simulink model "Six_DOF"  (R2017a)
settings: Solver=ode45  StartTime=0.0  StopTime=10  MaxStep=2.0  RelTol=1e-3
InitFcn:
  | initializeVariables
StopFcn:
  | postProcessResults
undefined symbols (not defined in the file): airplane, cl_fit, cm_fit, cx_fit, m
libraries: simulink_extras x5, aerolibasang x3, shared6dof x1
settings Model: Creator=Devansh  LastModifiedBy=Devansh
settings HardwareCC: ProdBitPerLong=64  ProdHWDeviceType=Intel->x86-64 (Mac OS X)

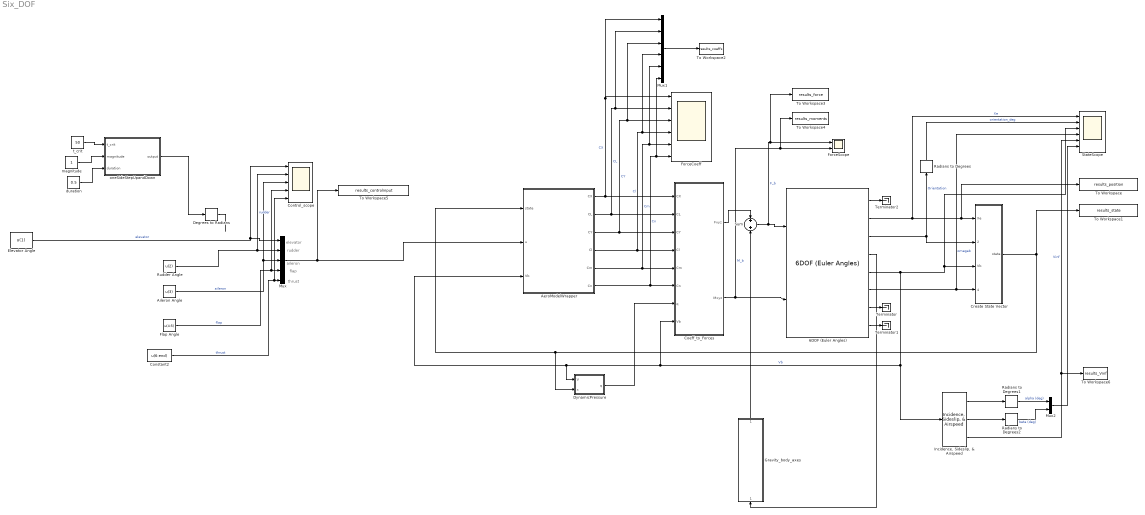
== system Six_DOF ==
  note: thrust
  note: flap
  note: aileron
  note: rudder
  note: elevator
  6DOF (Euler Angles) : shared6dof/6DOF (Euler Angles)  units=Metric (MKS)  mtype=Fixed  rep=Euler Angles  xme_0=initial_position  Vm_0=initial_velocity  eul_0=initial_orientation  pm_0=initial_rotation_rate  mass_0=m  mass_e=0.5  mass_f=2.0  inertia=inertia_matrix  inertia_e=eye(3)  inertia_f=2*eye(3)  k_quat=1.0  vre_flag=on  abi_flag=off
  AeroModelWrapper : Subsystem
  Aileron Angle : Constant  Value=u(3)
  Coeff_to_Forces : Subsystem  TreatAsAtomicUnit=on
  Constant2 : Constant  Value=u(6:end)
  Control_scope : Scope  NumInputPorts=5
  Create State Vector : Subsystem
  Degrees to Radians : simulink_extras/Transformations/Degrees to Radians
  DynamicPressure : MATLAB Function  TreatAsAtomicUnit=on
  Elevator Angle : Constant  Value=u(1)
  Flap Angle : Constant  Value=u(4:5)
  ForceCoeff : Scope  NumInputPorts=6
  ForceScope : Scope  NumInputPorts=2
  Gravity_body_axes : Subsystem
  "Incidence, Sideslip, & Airspeed" : aerolibasang/Incidence, Sideslip, & Airspeed
      settings: SourceProductName=Aerospace Blockset
  Mux : Mux  Inputs=5
  Mux1 : Mux  Inputs=6
  Mux2 : Mux  Inputs=2
  Radians to Degrees : simulink_extras/Transformations/Radians to Degrees
  Radians to Degrees1 : simulink_extras/Transformations/Radians to Degrees
  Radians to Degrees2 : simulink_extras/Transformations/Radians to Degrees
  Rudder Angle : Constant  Value=u(2)
  "StateScope " : Scope  NumInputPorts=6
  Sum : Sum  Inputs=+|+
  Terminator : Terminator
  Terminator1 : Terminator
  Terminator2 : Terminator
  To Workspace : ToWorkspace  VariableName=results_position  SaveFormat=Timeseries  SampleTime=-1
  To Workspace1 : ToWorkspace  VariableName=results_state  SaveFormat=Timeseries  SampleTime=-1
  To Workspace2 : ToWorkspace  VariableName=results_coeffs  SaveFormat=Timeseries  SampleTime=-1
  To Workspace3 : ToWorkspace  VariableName=results_force  SaveFormat=Timeseries  SampleTime=-1
  To Workspace4 : ToWorkspace  VariableName=results_moments  SaveFormat=Timeseries  SampleTime=-1
  To Workspace5 : ToWorkspace  VariableName=results_controlinput  SaveFormat=Timeseries  SampleTime=-1
  To Workspace6 : ToWorkspace  VariableName=results_Vinf  SaveFormat=Timeseries  SampleTime=-1
  duration : Constant  Value=0.5
  magnitude : Constant
  oneSideStepUpandDown : Subsystem
  t_crit : Constant  Value=50
  wires:
  AeroModelWrapper/1(CX) -> Coeff_to_Forces/1(CX), Mux1/1, ForceCoeff/1  "CX"
  AeroModelWrapper/3(CY) -> Coeff_to_Forces/3(CY), Mux1/3, ForceCoeff/3  "CY"
  AeroModelWrapper/2(CL) -> Coeff_to_Forces/2(CL), Mux1/2, ForceCoeff/2  "CL"
  AeroModelWrapper/4(Cl) -> Mux1/4, ForceCoeff/4, Coeff_to_Forces/4(Cl)  "Cl"
  AeroModelWrapper/5(Cm) -> Mux1/5, ForceCoeff/5, Coeff_to_Forces/5(Cm)  "Cm"
  AeroModelWrapper/6(Cn) -> Mux1/6, ForceCoeff/6, Coeff_to_Forces/6(Cn)  "Cn"
  Coeff_to_Forces/2(Mxyz) -> To Workspace4/1, ForceScope/2, 6DOF (Euler Angles)/2  "M_b"
  DynamicPressure/1(q) -> Coeff_to_Forces/7(q)
  6DOF (Euler Angles)/2 -> "StateScope "/1, To Workspace/1, Create State Vector/1(Xe)  "Xe"
  6DOF (Euler Angles)/3 -> Create State Vector/2(orientation), Radians to Degrees/1  "Orientation"
  6DOF (Euler Angles)/5 -> "StateScope "/3, Create State Vector/3(Vb), "Incidence, Sideslip, & Airspeed"/1, Coeff_to_Forces/8(Vb), AeroModelWrapper/3(Vb), DynamicPressure/1(V)  "Vb"
  6DOF (Euler Angles)/6 -> "StateScope "/4, Create State Vector/4(omega b)  "omegab"
  Flap Angle/1 -> Control_scope/4, Mux/4  "flap"
  Constant2/1 -> Control_scope/5, Mux/5  "thrust"
  "Incidence, Sideslip, & Airspeed"/3 -> "StateScope "/5, To Workspace6/1  "Vinf"
  "Incidence, Sideslip, & Airspeed"/1 -> Radians to Degrees1/1
  "Incidence, Sideslip, & Airspeed"/2 -> Radians to Degrees2/1
  Radians to Degrees/1 -> "StateScope "/2  "orientation_deg"
  Radians to Degrees1/1 -> Mux2/1  "alpha (deg)"
  Radians to Degrees2/1 -> Mux2/2  "beta (deg)"
  Coeff_to_Forces/1(Fxyz) -> Sum/1
  Sum/1 -> 6DOF (Euler Angles)/1, To Workspace3/1, ForceScope/1  "F_b"
  6DOF (Euler Angles)/4 -> Gravity_body_axes/1(Earth_to_body_rotation)
  Gravity_body_axes/1(Gravity_Body_coords) -> Sum/2
  Mux/1 -> To Workspace5/1, AeroModelWrapper/2(u)
  6DOF (Euler Angles)/7 -> Terminator/1
  6DOF (Euler Angles)/8 -> Terminator1/1
  6DOF (Euler Angles)/1 -> Terminator2/1
  Degrees to Radians/1 -> ?
  t_crit/1 -> oneSideStepUpandDown/1(t_crit)
  magnitude/1 -> oneSideStepUpandDown/2(magnitude)
  duration/1 -> oneSideStepUpandDown/3(duration)
  oneSideStepUpandDown/1(output) -> Degrees to Radians/1
  Elevator Angle/1 -> Control_scope/1, Mux/1  "elevator"
  Rudder Angle/1 -> Control_scope/2, Mux/2  "rudder"
  Aileron Angle/1 -> Control_scope/3, Mux/3  "aileron"
  Mux1/1 -> To Workspace2/1
  Create State Vector/1(state) -> To Workspace1/1, DynamicPressure/2(x), AeroModelWrapper/1(state)
  Mux2/1 -> "StateScope "/6

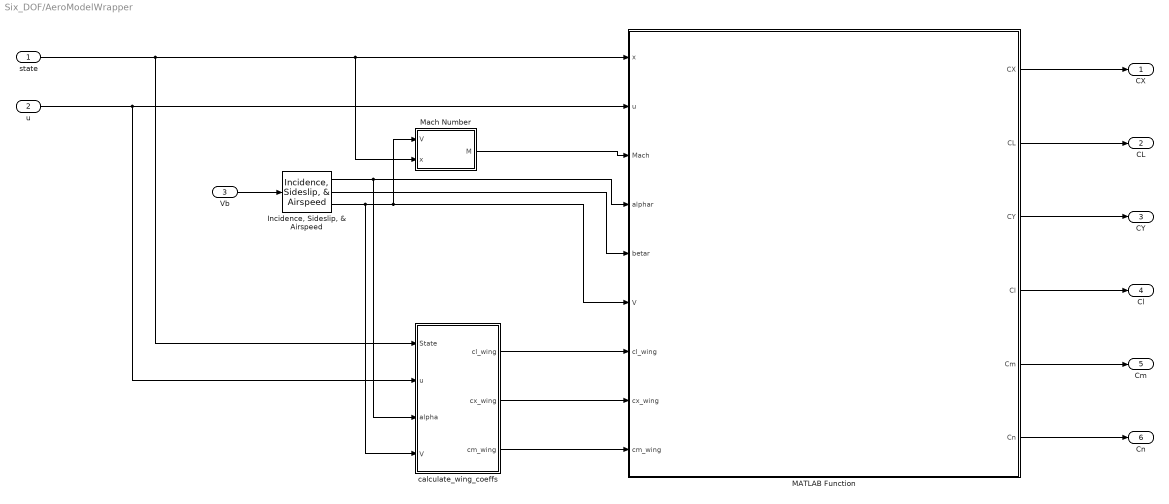
== system Six_DOF/AeroModelWrapper ==
  state : Inport
  u : Inport  Port=2
  Vb : Inport  Port=3
  "Incidence, Sideslip, & Airspeed" : aerolibasang/Incidence, Sideslip, & Airspeed
      settings: SourceProductName=Aerospace Blockset
  MATLAB Function : MATLAB Function  TreatAsAtomicUnit=on
  Mach Number : MATLAB Function  TreatAsAtomicUnit=on
  calculate_wing_coeffs : Subsystem
  CX : Outport
  CL : Outport  Port=2
  CY : Outport  Port=3
  Cl : Outport  Port=4
  Cm : Outport  Port=5
  Cn : Outport  Port=6
  wires:
  MATLAB Function/1(CX) -> CX/1
  MATLAB Function/2(CL) -> CL/1
  MATLAB Function/3(CY) -> CY/1
  MATLAB Function/4(Cl) -> Cl/1
  MATLAB Function/5(Cm) -> Cm/1
  MATLAB Function/6(Cn) -> Cn/1
  u/1 -> calculate_wing_coeffs/2(u), MATLAB Function/2(u)
  "Incidence, Sideslip, & Airspeed"/2 -> MATLAB Function/5(betar)
  "Incidence, Sideslip, & Airspeed"/1 -> calculate_wing_coeffs/3(alpha), MATLAB Function/4(alphar)
  "Incidence, Sideslip, & Airspeed"/3 -> calculate_wing_coeffs/4(V), Mach Number/1(V), MATLAB Function/6(V)
  Mach Number/1(M) -> MATLAB Function/3(Mach)
  Vb/1 -> "Incidence, Sideslip, & Airspeed"/1
  state/1 -> calculate_wing_coeffs/1(State), Mach Number/2(x), MATLAB Function/1(x)
  calculate_wing_coeffs/1(cl_wing) -> MATLAB Function/7(cl_wing)
  calculate_wing_coeffs/2(cx_wing) -> MATLAB Function/8(cx_wing)
  calculate_wing_coeffs/3(cm_wing) -> MATLAB Function/9(cm_wing)

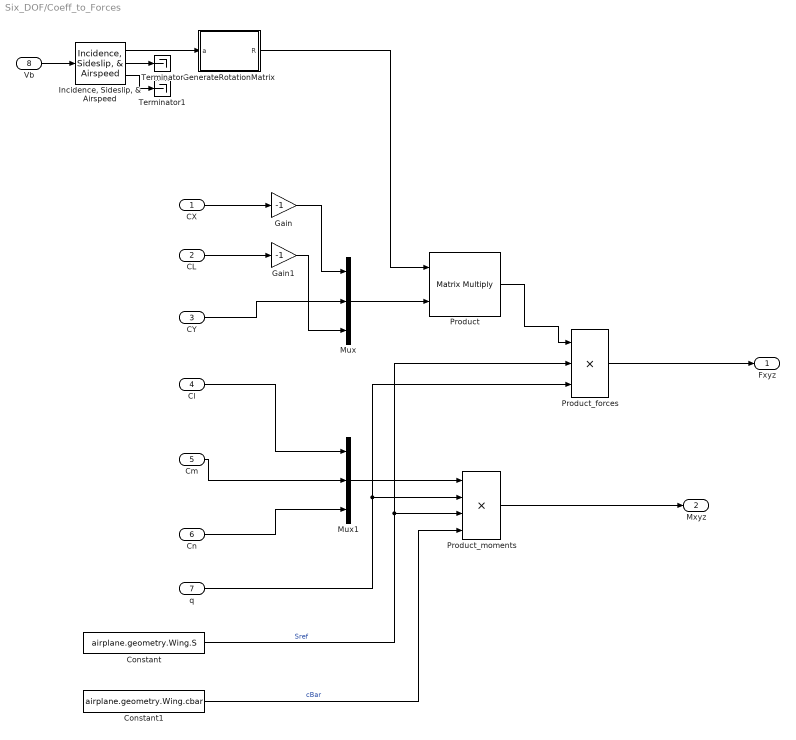
== system Six_DOF/Coeff_to_Forces ==
  CX : Inport
  CL : Inport  Port=2
  CY : Inport  Port=3
  Cl : Inport  Port=4
  Cm : Inport  Port=5
  Cn : Inport  Port=6
  q : Inport  Port=7
  Vb : Inport  Port=8
  Constant : Constant  Value=airplane.geometry.Wing.S
  Constant1 : Constant  Value=airplane.geometry.Wing.cbar
  Gain : Gain  Gain=-1
  Gain1 : Gain  Gain=-1
  GenerateRotationMatrix : MATLAB Function  TreatAsAtomicUnit=on
  "Incidence, Sideslip, & Airspeed" : aerolibasang/Incidence, Sideslip, & Airspeed
      settings: SourceProductName=Aerospace Blockset
  Mux : Mux  Inputs=3
  Mux1 : Mux  Inputs=3
  Product : Product  Multiplication=Matrix(*)
  Product_forces : Product  Inputs=3
  Product_moments : Product  Inputs=4
  Terminator : Terminator
  Terminator1 : Terminator
  Fxyz : Outport
  Mxyz : Outport  Port=2
  wires:
  CX/1 -> Gain/1
  CL/1 -> Gain1/1
  Gain/1 -> Mux/1
  Gain1/1 -> Mux/3
  CY/1 -> Mux/2
  Constant/1 -> Product_moments/3, Product_forces/2  "Sref"
  q/1 -> Product_forces/3, Product_moments/2
  Product_forces/1 -> Fxyz/1
  Mux1/1 -> Product_moments/1
  Cl/1 -> Mux1/1
  Cm/1 -> Mux1/2
  Cn/1 -> Mux1/3
  Constant1/1 -> Product_moments/4  "cBar"
  Product_moments/1 -> Mxyz/1
  Mux/1 -> Product/2
  GenerateRotationMatrix/1(R) -> Product/1
  Product/1 -> Product_forces/1
  Vb/1 -> "Incidence, Sideslip, & Airspeed"/1
  "Incidence, Sideslip, & Airspeed"/1 -> GenerateRotationMatrix/1(a)
  "Incidence, Sideslip, & Airspeed"/2 -> Terminator/1
  "Incidence, Sideslip, & Airspeed"/3 -> Terminator1/1

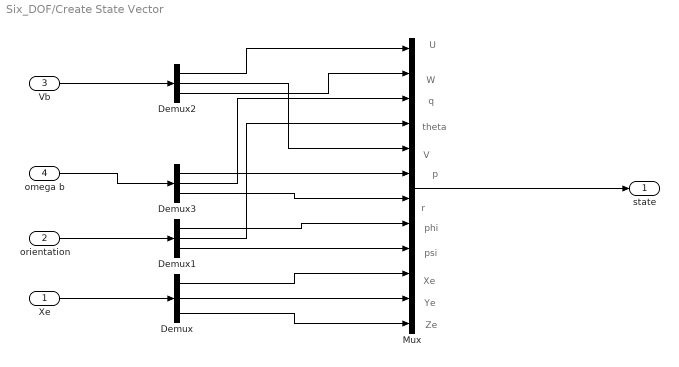
== system Six_DOF/Create State Vector ==
  note: Ze
  note: Ye
  note: Xe
  note: psi
  note: phi
  note: r
  note: p
  note: V
  note: theta
  note: q
  note: W
  note: U
  Xe : Inport
  orientation : Inport  Port=2
  Vb : Inport  Port=3
  omega b : Inport  Port=4
  Demux{,1..3} (4 alike) : Demux  Outputs=3
  Mux : Mux  Inputs=12
  state : Outport
  wires:
  Demux2/1 -> Mux/1
  Demux2/2 -> Mux/5
  Vb/1 -> Demux2/1
  Demux1/1 -> Mux/8
  Demux/1 -> Mux/10
  Demux/3 -> Mux/12
  Xe/1 -> Demux/1
  orientation/1 -> Demux1/1
  Mux/1 -> state/1
  Demux3/1 -> Mux/6
  Demux1/3 -> Mux/9
  Demux/2 -> Mux/11
  Demux3/2 -> Mux/3
  Demux1/2 -> Mux/4
  Demux2/3 -> Mux/2
  Demux3/3 -> Mux/7
  omega b/1 -> Demux3/1

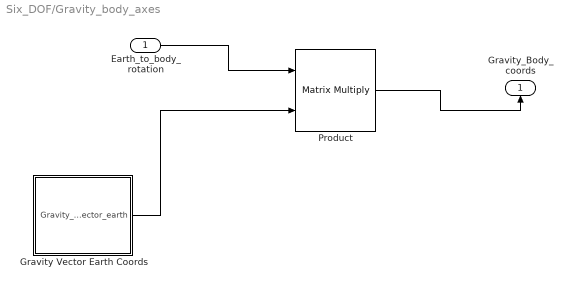
== system Six_DOF/Gravity_body_axes ==
  Earth_to_body_rotation : Inport
  Gravity Vector Earth Coords : Subsystem
  Product : Product  Multiplication=Matrix(*)
  Gravity_Body_coords : Outport
  wires:
  Earth_to_body_rotation/1 -> Product/1
  Gravity Vector Earth Coords/1("Gravity_vector_earth ") -> Product/2
  Product/1 -> Gravity_Body_coords/1

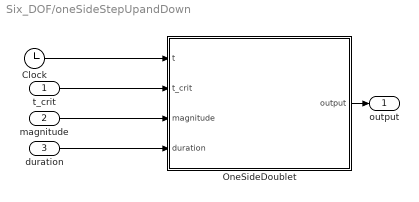
== system Six_DOF/oneSideStepUpandDown ==
  t_crit : Inport
  magnitude : Inport  Port=2
  duration : Inport  Port=3
  Clock : Clock
      settings: Decimation=100
  OneSideDoublet : MATLAB Function  TreatAsAtomicUnit=on
  output : Outport
  wires:
  duration/1 -> OneSideDoublet/4(duration)
  t_crit/1 -> OneSideDoublet/2(t_crit)
  OneSideDoublet/1(output) -> output/1
  Clock/1 -> OneSideDoublet/1(t)
  magnitude/1 -> OneSideDoublet/3(magnitude)

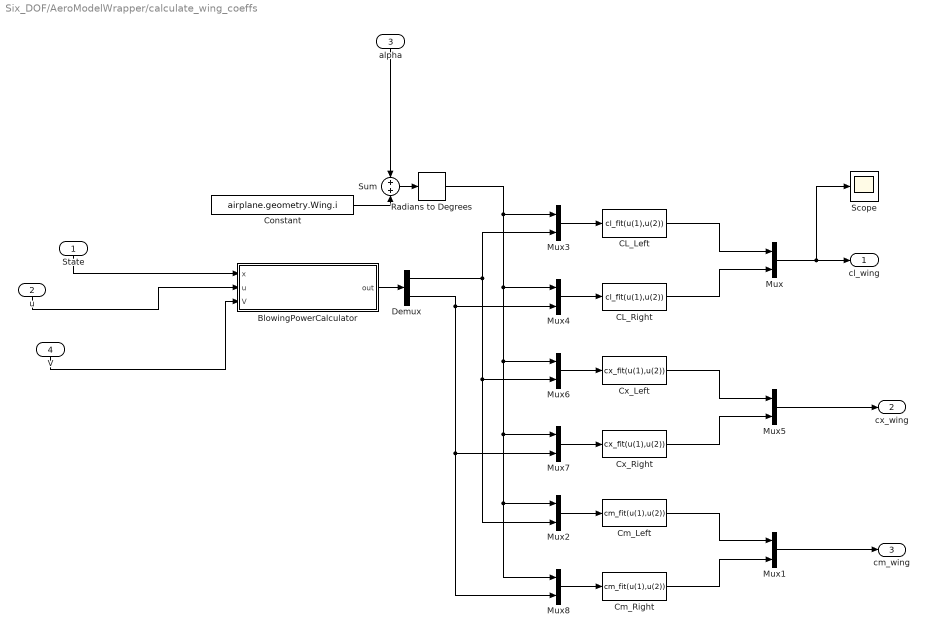
== system Six_DOF/AeroModelWrapper/calculate_wing_coeffs ==
  State : Inport
  u : Inport  Port=2
  alpha : Inport  Port=3
  V : Inport  Port=4
  BlowingPowerCalculator : MATLAB Function  TreatAsAtomicUnit=on
  CL_Left : MATLABFcn  MATLABFcn=cl_fit(u(1),u(2))  OutputDimensions=1
  CL_Right : MATLABFcn  MATLABFcn=cl_fit(u(1),u(2))  OutputDimensions=1
  Cm_Left : MATLABFcn  MATLABFcn=cm_fit(u(1),u(2))  OutputDimensions=1
  Cm_Right : MATLABFcn  MATLABFcn=cm_fit(u(1),u(2))  OutputDimensions=1
  Constant : Constant  Value=airplane.geometry.Wing.i
  Cx_Left : MATLABFcn  MATLABFcn=cx_fit(u(1),u(2))  OutputDimensions=1
  Cx_Right : MATLABFcn  MATLABFcn=cx_fit(u(1),u(2))  OutputDimensions=1
  Demux : Demux  Outputs=2
  Mux{,1..8} (9 alike) : Mux  Inputs=2
  Radians to Degrees : simulink_extras/Transformations/Radians to Degrees
  Scope : Scope
  Sum : Sum  Inputs=+|+
  cl_wing : Outport
  cx_wing : Outport  Port=2
  cm_wing : Outport  Port=3
  wires:
  State/1 -> BlowingPowerCalculator/1(x)
  alpha/1 -> Sum/1
  u/1 -> BlowingPowerCalculator/2(u)
  Mux/1 -> Scope/1, cl_wing/1
  Constant/1 -> Sum/2
  Sum/1 -> Radians to Degrees/1
  Mux1/1 -> cm_wing/1
  BlowingPowerCalculator/1(out) -> Demux/1
  V/1 -> BlowingPowerCalculator/3(V)
  Mux3/1 -> CL_Left/1
  CL_Left/1 -> Mux/1
  Mux4/1 -> CL_Right/1
  CL_Right/1 -> Mux/2
  Cx_Left/1 -> Mux5/1
  Cx_Right/1 -> Mux5/2
  Mux5/1 -> cx_wing/1
  Mux7/1 -> Cx_Right/1
  Mux6/1 -> Cx_Left/1
  Mux2/1 -> Cm_Left/1
  Cm_Left/1 -> Mux1/1
  Cm_Right/1 -> Mux1/2
  Mux8/1 -> Cm_Right/1
  Demux/1 -> Mux2/2, Mux6/2, Mux3/2
  Demux/2 -> Mux4/2, Mux8/2, Mux7/2
  Radians to Degrees/1 -> Mux6/1, Mux2/1, Mux8/1, Mux7/1, Mux4/1, Mux3/1

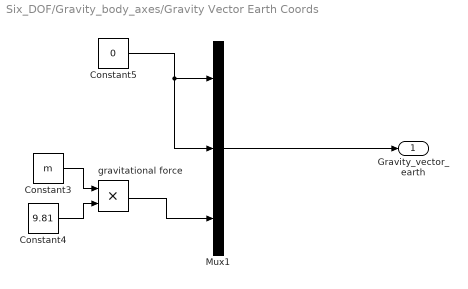
== system Six_DOF/Gravity_body_axes/Gravity Vector Earth Coords ==
  Constant3 : Constant  Value=m
  Constant4 : Constant  Value=9.81
  Constant5 : Constant  Value=0
  Mux1 : Mux  Inputs=3
  gravitational force : Product
  "Gravity_vector_earth " : Outport
  wires:
  Constant4/1 -> gravitational force/2
  Constant3/1 -> gravitational force/1
  Constant5/1 -> Mux1/2, Mux1/1
  gravitational force/1 -> Mux1/3
  Mux1/1 -> "Gravity_vector_earth "/1

== matlab function Six_DOF/DynamicPressure ==
  data: V input; q output; x input
function q = fcn(V,x)
%calculates the dynamic pressure using the flight speed and airspeed

h=-x(12); %extract the height

[~, ~, rho, ~, ~, ~, ~, ~] = int_std_atm(h);


q = 0.5*rho*norm(V)^2;


end

== matlab function Six_DOF/AeroModelWrapper/MATLAB Function ==
  data: x input; u input; CX output; Mach input; alphar input; betar input; V input; CL output; CY output; Cl output; Cm output; Cn output; cl_wing input; cx_wing input; cm_wing input
	function [CX,CL,CY,Cl,Cm,Cn] = AeroModelSSTOL(x,u,Mach,alphar,betar,V, cl_wing, cx_wing, cm_wing)
%	SSTOL Aero Model
%   x(1) = u_b          Body axis u velocity, m/s
%   x(2) = w_b          Body axis w velocity, m/s
%   x(3) = q            Pitch rate, rad/s
%   x(4) = theta        Pitch euler angle, rad
%   x(5) = v_b          Body axis v velocity, m/s
%   x(6) = p            Roll rate, rad/s
%   x(7) = r            Yaw rate, rad/s
%   x(8) = phi          Roll euler angle, rad
%   x(9) = psi          Yaw euler angle, rad
%   x(10) = xe          North position, Earth frame, m
%   x(11) = ye          East position, Earth frame, m
%   x(12) = ze =-h      Negative of altitude, Earth frame, m

%   u(1) = elevator deflection, rad, positive trailing edge down
%   u(2) = rudder deflection, rad, positive trailing edge down
%   u(3) = aileron deflection, rad, positive left trailing edge down
%   u(4) = left flap deflection, rad, positive trailing edge down
%   u(5) = right flap deflection, rad, positive trailing edge down
%   u(6:end) = u_t, thrust control vector, 0-1

%   u_thrust(1) = left blowing throttle, 0-1
%   u_thrust(2) = right blowing throttle, 0-1
%   u_thrust(3) = left thruster throttle, 0-1
%   u_thrust(4) = right thruster throttle, 0-1

%	Inertial, Geometric, and Aerodynamic Properties
%   *** STOL_Input.m must first be run to save Airplane.mat***
	

    A=coder.load('./SSTOL_Aero_Model/Airplane.mat');
    airplane=A.airplane;
    
    %Handy variable shorthands
    i_w = airplane.geometry.Wing.i;
    i_t = airplane.geometry.Htail.i;
    cbar = airplane.geometry.Wing.cbar;
    e = airplane.aero.Wing.e; %TODO: Make this a function of delta_f, etc.
    AR = airplane.geometry.Wing.AR;
    clat = airplane.aero.Htail.cla;
    Sh = airplane.geometry.Htail.S;
    Sv = airplane.geometry.Vtail.S;
    Sw = airplane.geometry.Wing.S;
    lh = airplane.geometry.Htail.l;
    lv = airplane.geometry.Vtail.l;
    b  = airplane.geometry.Wing.b;
    Vv = Sv/Sw*lv/b;
    Vh = Sh/Sw*lh/cbar;
    tau_h = airplane.aero.Htail.tau;
    x_cg = airplane.weights.xcg;
    x_acw = airplane.aero.Wing.x_ac;
    
    alt = -x(12);
    
    rad2deg = 180/pi;
    
    alpha_w     = alphar + i_w;
	a_w_deg	=	(alpha_w)*rad2deg;
    
    %Thrust Control vector
    u_t = u(6:end);
    d_BL = u_t(1);
    d_BR = u_t(2);
    d_TL = u_t(3);
    d_TR = u_t(4);

%   Blowing and Thrust Calculations
%   ====================================
    [dCJ_BL, ~, CT_BL] = propulsor_perf(d_BL, airplane.propulsion.left_blower, cbar, alt, V);
    [dCJ_BR, ~, CT_BR] = propulsor_perf(d_BR, airplane.propulsion.right_blower, cbar, alt, V);
    [~, T_L, CT_CL] = propulsor_perf(d_TL, airplane.propulsion.left_cruiser, cbar, alt, V);
    [~, T_R, CT_CR] = propulsor_perf(d_TR, airplane.propulsion.right_cruiser, cbar, alt, V);
    
%	CL Calculations 
%	====================================

    %Wing Lift Coefficient
    %C_L_wing
    %Currently this interpolator is only for 40deg flaps; any
    %flap changes are ignored.

    cl_left = cl_wing(1);
    cl_right = cl_wing(2); %if there is a two element vector, it takes the second, if its a scalar, it takes the only value.
    
    %cl_left = cl_fit(round(a_w_deg), round(dCJ_BL))
    %cl_right = cl_fit(round(a_w_deg), round(dCJ_BR))

    
    CLw = .9*(cl_left + cl_right)/2;
    
    %Tail Lift Coefficient
    %C_L_ht
    eta_h = 1; %Update with better method of estimating tail dynamic pressure ratio
    eps = 2*CLw/(pi*e*AR); %May want to use M&S method here instead
    a_h = (alphar+i_t-eps);
    
    eta = clat/(2*pi);
    sweep_h = airplane.geometry.Htail.sweep;
    CLah = (2*pi*AR)/(2+sqrt(4*(AR/eta)^2*(1+tan(sweep_h)^2)));
    CLt = CLah*a_h*Sh/Sw*eta_h;
    %Elevator and Pitch Rate effects
    CLde = airplane.stability.CLde;
    CLde_check = Sh/Sw*CLah*tau_h;
    CLde = CLde_check; %Very different drom JVL; need to debug
    CLq = airplane.stability.CLq;
    CLq_check = -2*Vh*CLah;
    CLq = CLq_check; %Very different drom JVL; need to debug
    CL = CLw + CLah*a_h + CLq*x(3) + CLde*u(1);

%	CX Calculations 
%	====================================
    cx_left = cx_wing(1);
    cx_right = cx_wing(2);
    
    CXw = (cx_left+cx_right)/2;
    CDi = CLw^2/(pi*AR*e+(CT_BL+CT_BR));
    CDp = .03;  %Placeholder, this has little effect on the high-lift cases
    
    CX = CXw + CDi + CDp - CT_CL - CT_CR;

%	Cm Calculations 
%	====================================    
    cm_left     = cm_wing(1);
    cm_right    = cm_wing(2);
    
    Cmw = (cm_left + cm_right)/2;
    Cmh = -Vh*eta_h*CLah*a_h;
    
    Cmde = airplane.stability.Cmde;
    Cmq = airplane.stability.Cmq;
    
    Cmaf = 0; %Negelect fuselage contributions for now
    Cmf = Cmaf*alphar;
    
    Cm = CLw*(x_cg-x_acw)/cbar + Cmw + Cmh + Cmf + Cmde*u(1) + Cmq*x(3);
    
    	
%	Current Lateral-Directional Characteristics
%	===========================================
%	Cl Calculations 
%	==================================== 
%	Rolling Moment Coefficient

	%Cl      =	(ClBr*betar + CldRr*u(2)) + Clrr * x(7) + Clpr * x(6) ...
    %            + (CldAr*u(3));% + CldASr*u(5));
									% Total Rolling-Moment Coefficient
    Cl = 0;

%	CY Calculations 
%	==================================== 
%	Side-Force Coefficient
	%CY	=	(CYBr*betar + CYdRr*u(2)) + (CYdAr*u(3));% + CYdASr*u(5));
									% Total Side-Force Coefficient
    CY = 0;
%	Cn Calculations 
%	====================================                                     
%	Yawing Moment Coefficient
	%Cn	=	(CnBr*betar + CndRr*u(2)) + Cnrr * x(7) + Cnpr * x(6) ...
	%		+ (CndAr*u(3));% + CndASr*u(5));
									% Total Yawing-Moment Coefficient
    Cn = 0;

== matlab function Six_DOF/AeroModelWrapper/Mach Number ==
  data: V input; M output; x input
function M = fcn(V,x)
%calculates the mach number

[~, ~, ~, a, ~, ~, ~, ~] = int_std_atm(-x(12));

M = norm(V)/a;

== matlab function Six_DOF/Coeff_to_Forces/GenerateRotationMatrix ==
  data: a input; R output
function R = rotationMatrix(a)

R = [cos(a), 0, -sin(a); 0, 1, 0; sin(a), 0, cos(a)];

== matlab function Six_DOF/oneSideStepUpandDown/OneSideDoublet ==
  data: t input; output output; t_crit input; magnitude input; duration input
function output = oneSideDoublet(t,t_crit,magnitude,duration)

if t > t_crit && t<(t_crit + duration)
    output = magnitude;
else
    output = 0;
end

== matlab function Six_DOF/AeroModelWrapper/calculate_wing_coeffs/BlowingPowerCalculator ==
  data: x input; u input; out output; V input
function out = fcn(x,u,V)
%% this function gets the blowing power levels

A=coder.load('./SSTOL_Aero_Model/Airplane.mat');
airplane=A.airplane;

%Handy variable shorthands

cbar = airplane.geometry.Wing.cbar;

alt = -x(12);

%Thrust Control vector
u_t = u(6:end);
d_BL = u_t(1);
d_BR = u_t(2);

%   Blowing and Thrust Calculations
%   ====================================
[dCJ_BL, ~, ~] = propulsor_perf(d_BL, airplane.propulsion.left_blower, cbar, alt, V);
[dCJ_BR, ~, ~] = propulsor_perf(d_BR, airplane.propulsion.right_blower, cbar, alt, V);


out = zeros(2,1);

out(1) = dCJ_BL;
out(2) = dCJ_BR;
end
